simulink model "ENV_old_working"  (R2024b)
settings: Solver=FixedStepDiscrete  StartTime=0.0  StopTime=1  FixedStep=0.001  RelTol=1e-3  EnableMultiTasking=on
libraries: stm32blockslib x68, canmsglib x32, stm32f4xxblockslib x20, simulink x8
(part 3 of 4)

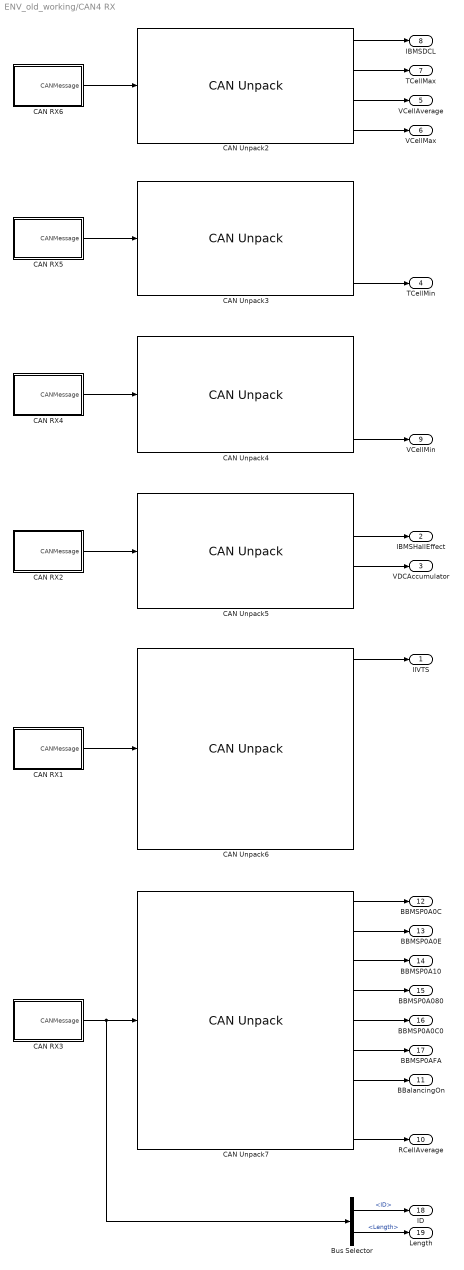
== system ENV_old_working/CAN4 RX ==
  Bus Selector : BusSelector  OutputSignals=ID,Length
  CAN RX1 : Subsystem  mask{SPIModuleSelect=SPI1, Port_Select=GPIOC, Pin=5, PortName=GPIOC, PinNumber=4}
      mask prompts: SPIModuleSelect "SPI Module"; Port_Select "CS Port"; Pin "CS Pin"; PortName "INT Port"; PinNumber "INT Pin"
      mask TypeOptions SPIModuleSelect:
      | Enabled
      | Subsystem/SPI Controller Transfer7/SPIModuleSelect
      mask TypeOptions Port_Select:
      | Enabled
      | Subsystem/SPI Controller Transfer7/Port_Select
      mask TypeOptions Pin:
      | Enabled
      | Subsystem/SPI Controller Transfer7/Pin
      mask TypeOptions PortName: Digital Port Read5/PortName
      mask TypeOptions PinNumber: Digital Port Read5/PinNumber
      mask DialogControl DescTextVar Prompt: Read RX buffer when the INT pin is pulled low. Outputs a CANMessage type to be fed into a CAN unpack
      mask Display:
      | %port_label('output', 1, 'CANMessage');
      | 
      | text(0.05, 0.5, '' + string(get_param(gcb,'SPIModuleSelect')), HorizontalAlignment = 'left');
      | text(0.05, 0.85, 'CS ' + string(get_param(gcb,'Port_Select')) + ' Pin ' + string(get_param(gcb,'Pin')), HorizontalAlignment = 'left');
      | 
      | 
      | text(0.05, 0.15, 'INT ' + string(get_param(gcb,'PortName')) + ' Pin ' + string(get_param(gcb,'PinNumber')), HorizontalAlignment = 'left');
      | %text(0.05, 0.15, 'INT Pin ' + string(get_param(gcb,'PinNumber')), HorizontalAlignment = 'left');
      | 
      | 
      | % OBR logo
      | pos = get_param(gcb, 'Position');
      | blockAspect = (pos(3)-pos(1)) / (pos(4)-pos(2));
      | 
      | % fit(img, m, cx, cy): m = fraction of block the image occupies,
      | % (cx,cy) = center point in normalized 0-1 coords
      | fit = @(img,m,cx,cy) [ ...
      |     cx - m*min(1,(size(img,2)/size(img,1))/blockAspect)/2, ...
      |     cy - m*min(1,blockAspect/(size(img,2)/size(img,1)))/2, ...
      |     m*min(1,(size(img,2)/size(img,1))/blockAspect), ...
      |     m*min(1,blockAspect/(size(img,2)/size(img,1))) ];
      | 
      | ud = get_param(gcb, 'UserData');
      | 
      | image(ud.mcplogo, fit(ud.mcplogo, 0.3, 0.85, 0.5));
      | image(ud.obrlogo, fit(ud.obrlogo, 0.5, 0.5, 0.5));
  CAN RX2 : Subsystem  mask{SPIModuleSelect=SPI1, Port_Select=GPIOC, Pin=5, PortName=GPIOC, PinNumber=4}
      mask prompts: SPIModuleSelect "SPI Module"; Port_Select "CS Port"; Pin "CS Pin"; PortName "INT Port"; PinNumber "INT Pin"
      mask TypeOptions SPIModuleSelect:
      | Enabled
      | Subsystem/SPI Controller Transfer7/SPIModuleSelect
      mask TypeOptions Port_Select:
      | Enabled
      | Subsystem/SPI Controller Transfer7/Port_Select
      mask TypeOptions Pin:
      | Enabled
      | Subsystem/SPI Controller Transfer7/Pin
      mask TypeOptions PortName: Digital Port Read5/PortName
      mask TypeOptions PinNumber: Digital Port Read5/PinNumber
      mask DialogControl DescTextVar Prompt: Read RX buffer when the INT pin is pulled low. Outputs a CANMessage type to be fed into a CAN unpack
      mask Display:
      | %port_label('output', 1, 'CANMessage');
      | 
      | text(0.05, 0.5, '' + string(get_param(gcb,'SPIModuleSelect')), HorizontalAlignment = 'left');
      | text(0.05, 0.85, 'CS ' + string(get_param(gcb,'Port_Select')) + ' Pin ' + string(get_param(gcb,'Pin')), HorizontalAlignment = 'left');
      | 
      | 
      | text(0.05, 0.15, 'INT ' + string(get_param(gcb,'PortName')) + ' Pin ' + string(get_param(gcb,'PinNumber')), HorizontalAlignment = 'left');
      | %text(0.05, 0.15, 'INT Pin ' + string(get_param(gcb,'PinNumber')), HorizontalAlignment = 'left');
      | 
      | 
      | % OBR logo
      | pos = get_param(gcb, 'Position');
      | blockAspect = (pos(3)-pos(1)) / (pos(4)-pos(2));
      | 
      | % fit(img, m, cx, cy): m = fraction of block the image occupies,
      | % (cx,cy) = center point in normalized 0-1 coords
      | fit = @(img,m,cx,cy) [ ...
      |     cx - m*min(1,(size(img,2)/size(img,1))/blockAspect)/2, ...
      |     cy - m*min(1,blockAspect/(size(img,2)/size(img,1)))/2, ...
      |     m*min(1,(size(img,2)/size(img,1))/blockAspect), ...
      |     m*min(1,blockAspect/(size(img,2)/size(img,1))) ];
      | 
      | ud = get_param(gcb, 'UserData');
      | 
      | image(ud.mcplogo, fit(ud.mcplogo, 0.3, 0.85, 0.5));
      | image(ud.obrlogo, fit(ud.obrlogo, 0.5, 0.5, 0.5));
  CAN RX3 : Subsystem  mask{SPIModuleSelect=SPI1, Port_Select=GPIOC, Pin=5, PortName=GPIOC, PinNumber=4}
      mask prompts: SPIModuleSelect "SPI Module"; Port_Select "CS Port"; Pin "CS Pin"; PortName "INT Port"; PinNumber "INT Pin"
      mask TypeOptions SPIModuleSelect:
      | Enabled
      | Subsystem/SPI Controller Transfer7/SPIModuleSelect
      mask TypeOptions Port_Select:
      | Enabled
      | Subsystem/SPI Controller Transfer7/Port_Select
      mask TypeOptions Pin:
      | Enabled
      | Subsystem/SPI Controller Transfer7/Pin
      mask TypeOptions PortName: Digital Port Read5/PortName
      mask TypeOptions PinNumber: Digital Port Read5/PinNumber
      mask DialogControl DescTextVar Prompt: Read RX buffer when the INT pin is pulled low. Outputs a CANMessage type to be fed into a CAN unpack
      mask Display:
      | %port_label('output', 1, 'CANMessage');
      | 
      | text(0.05, 0.5, '' + string(get_param(gcb,'SPIModuleSelect')), HorizontalAlignment = 'left');
      | text(0.05, 0.85, 'CS ' + string(get_param(gcb,'Port_Select')) + ' Pin ' + string(get_param(gcb,'Pin')), HorizontalAlignment = 'left');
      | 
      | 
      | text(0.05, 0.15, 'INT ' + string(get_param(gcb,'PortName')) + ' Pin ' + string(get_param(gcb,'PinNumber')), HorizontalAlignment = 'left');
      | %text(0.05, 0.15, 'INT Pin ' + string(get_param(gcb,'PinNumber')), HorizontalAlignment = 'left');
      | 
      | 
      | % OBR logo
      | pos = get_param(gcb, 'Position');
      | blockAspect = (pos(3)-pos(1)) / (pos(4)-pos(2));
      | 
      | % fit(img, m, cx, cy): m = fraction of block the image occupies,
      | % (cx,cy) = center point in normalized 0-1 coords
      | fit = @(img,m,cx,cy) [ ...
      |     cx - m*min(1,(size(img,2)/size(img,1))/blockAspect)/2, ...
      |     cy - m*min(1,blockAspect/(size(img,2)/size(img,1)))/2, ...
      |     m*min(1,(size(img,2)/size(img,1))/blockAspect), ...
      |     m*min(1,blockAspect/(size(img,2)/size(img,1))) ];
      | 
      | ud = get_param(gcb, 'UserData');
      | 
      | image(ud.mcplogo, fit(ud.mcplogo, 0.3, 0.85, 0.5));
      | image(ud.obrlogo, fit(ud.obrlogo, 0.5, 0.5, 0.5));
  CAN RX4 : Subsystem  mask{SPIModuleSelect=SPI1, Port_Select=GPIOC, Pin=5, PortName=GPIOC, PinNumber=4}
      mask prompts: SPIModuleSelect "SPI Module"; Port_Select "CS Port"; Pin "CS Pin"; PortName "INT Port"; PinNumber "INT Pin"
      mask TypeOptions SPIModuleSelect:
      | Enabled
      | Subsystem/SPI Controller Transfer7/SPIModuleSelect
      mask TypeOptions Port_Select:
      | Enabled
      | Subsystem/SPI Controller Transfer7/Port_Select
      mask TypeOptions Pin:
      | Enabled
      | Subsystem/SPI Controller Transfer7/Pin
      mask TypeOptions PortName: Digital Port Read5/PortName
      mask TypeOptions PinNumber: Digital Port Read5/PinNumber
      mask DialogControl DescTextVar Prompt: Read RX buffer when the INT pin is pulled low. Outputs a CANMessage type to be fed into a CAN unpack
      mask Display:
      | %port_label('output', 1, 'CANMessage');
      | 
      | text(0.05, 0.5, '' + string(get_param(gcb,'SPIModuleSelect')), HorizontalAlignment = 'left');
      | text(0.05, 0.85, 'CS ' + string(get_param(gcb,'Port_Select')) + ' Pin ' + string(get_param(gcb,'Pin')), HorizontalAlignment = 'left');
      | 
      | 
      | text(0.05, 0.15, 'INT ' + string(get_param(gcb,'PortName')) + ' Pin ' + string(get_param(gcb,'PinNumber')), HorizontalAlignment = 'left');
      | %text(0.05, 0.15, 'INT Pin ' + string(get_param(gcb,'PinNumber')), HorizontalAlignment = 'left');
      | 
      | 
      | % OBR logo
      | pos = get_param(gcb, 'Position');
      | blockAspect = (pos(3)-pos(1)) / (pos(4)-pos(2));
      | 
      | % fit(img, m, cx, cy): m = fraction of block the image occupies,
      | % (cx,cy) = center point in normalized 0-1 coords
      | fit = @(img,m,cx,cy) [ ...
      |     cx - m*min(1,(size(img,2)/size(img,1))/blockAspect)/2, ...
      |     cy - m*min(1,blockAspect/(size(img,2)/size(img,1)))/2, ...
      |     m*min(1,(size(img,2)/size(img,1))/blockAspect), ...
      |     m*min(1,blockAspect/(size(img,2)/size(img,1))) ];
      | 
      | ud = get_param(gcb, 'UserData');
      | 
      | image(ud.mcplogo, fit(ud.mcplogo, 0.3, 0.85, 0.5));
      | image(ud.obrlogo, fit(ud.obrlogo, 0.5, 0.5, 0.5));
  CAN RX5 : Subsystem  mask{SPIModuleSelect=SPI1, Port_Select=GPIOC, Pin=5, PortName=GPIOC, PinNumber=4}
      mask prompts: SPIModuleSelect "SPI Module"; Port_Select "CS Port"; Pin "CS Pin"; PortName "INT Port"; PinNumber "INT Pin"
      mask TypeOptions SPIModuleSelect:
      | Enabled
      | Subsystem/SPI Controller Transfer7/SPIModuleSelect
      mask TypeOptions Port_Select:
      | Enabled
      | Subsystem/SPI Controller Transfer7/Port_Select
      mask TypeOptions Pin:
      | Enabled
      | Subsystem/SPI Controller Transfer7/Pin
      mask TypeOptions PortName: Digital Port Read5/PortName
      mask TypeOptions PinNumber: Digital Port Read5/PinNumber
      mask DialogControl DescTextVar Prompt: Read RX buffer when the INT pin is pulled low. Outputs a CANMessage type to be fed into a CAN unpack
      mask Display:
      | %port_label('output', 1, 'CANMessage');
      | 
      | text(0.05, 0.5, '' + string(get_param(gcb,'SPIModuleSelect')), HorizontalAlignment = 'left');
      | text(0.05, 0.85, 'CS ' + string(get_param(gcb,'Port_Select')) + ' Pin ' + string(get_param(gcb,'Pin')), HorizontalAlignment = 'left');
      | 
      | 
      | text(0.05, 0.15, 'INT ' + string(get_param(gcb,'PortName')) + ' Pin ' + string(get_param(gcb,'PinNumber')), HorizontalAlignment = 'left');
      | %text(0.05, 0.15, 'INT Pin ' + string(get_param(gcb,'PinNumber')), HorizontalAlignment = 'left');
      | 
      | 
      | % OBR logo
      | pos = get_param(gcb, 'Position');
      | blockAspect = (pos(3)-pos(1)) / (pos(4)-pos(2));
      | 
      | % fit(img, m, cx, cy): m = fraction of block the image occupies,
      | % (cx,cy) = center point in normalized 0-1 coords
      | fit = @(img,m,cx,cy) [ ...
      |     cx - m*min(1,(size(img,2)/size(img,1))/blockAspect)/2, ...
      |     cy - m*min(1,blockAspect/(size(img,2)/size(img,1)))/2, ...
      |     m*min(1,(size(img,2)/size(img,1))/blockAspect), ...
      |     m*min(1,blockAspect/(size(img,2)/size(img,1))) ];
      | 
      | ud = get_param(gcb, 'UserData');
      | 
      | image(ud.mcplogo, fit(ud.mcplogo, 0.3, 0.85, 0.5));
      | image(ud.obrlogo, fit(ud.obrlogo, 0.5, 0.5, 0.5));
  CAN RX6 : Subsystem  mask{SPIModuleSelect=SPI1, Port_Select=GPIOC, Pin=5, PortName=GPIOC, PinNumber=4}
      mask prompts: SPIModuleSelect "SPI Module"; Port_Select "CS Port"; Pin "CS Pin"; PortName "INT Port"; PinNumber "INT Pin"
      mask TypeOptions SPIModuleSelect:
      | Enabled
      | Subsystem/SPI Controller Transfer7/SPIModuleSelect
      mask TypeOptions Port_Select:
      | Enabled
      | Subsystem/SPI Controller Transfer7/Port_Select
      mask TypeOptions Pin:
      | Enabled
      | Subsystem/SPI Controller Transfer7/Pin
      mask TypeOptions PortName: Digital Port Read5/PortName
      mask TypeOptions PinNumber: Digital Port Read5/PinNumber
      mask DialogControl DescTextVar Prompt: Read RX buffer when the INT pin is pulled low. Outputs a CANMessage type to be fed into a CAN unpack
      mask Display:
      | %port_label('output', 1, 'CANMessage');
      | 
      | text(0.05, 0.5, '' + string(get_param(gcb,'SPIModuleSelect')), HorizontalAlignment = 'left');
      | text(0.05, 0.85, 'CS ' + string(get_param(gcb,'Port_Select')) + ' Pin ' + string(get_param(gcb,'Pin')), HorizontalAlignment = 'left');
      | 
      | 
      | text(0.05, 0.15, 'INT ' + string(get_param(gcb,'PortName')) + ' Pin ' + string(get_param(gcb,'PinNumber')), HorizontalAlignment = 'left');
      | %text(0.05, 0.15, 'INT Pin ' + string(get_param(gcb,'PinNumber')), HorizontalAlignment = 'left');
      | 
      | 
      | % OBR logo
      | pos = get_param(gcb, 'Position');
      | blockAspect = (pos(3)-pos(1)) / (pos(4)-pos(2));
      | 
      | % fit(img, m, cx, cy): m = fraction of block the image occupies,
      | % (cx,cy) = center point in normalized 0-1 coords
      | fit = @(img,m,cx,cy) [ ...
      |     cx - m*min(1,(size(img,2)/size(img,1))/blockAspect)/2, ...
      |     cy - m*min(1,blockAspect/(size(img,2)/size(img,1)))/2, ...
      |     m*min(1,(size(img,2)/size(img,1))/blockAspect), ...
      |     m*min(1,blockAspect/(size(img,2)/size(img,1))) ];
      | 
      | ud = get_param(gcb, 'UserData');
      | 
      | image(ud.mcplogo, fit(ud.mcplogo, 0.3, 0.85, 0.5));
      | image(ud.obrlogo, fit(ud.obrlogo, 0.5, 0.5, 0.5));
  CAN Unpack2 : canmsglib/CAN Unpack  CANdbFile=C:\Users\Will\Desktop\OBR\Embedded\VCUSTM32\Controls\CAN\BMS\26.06.18_CAN4.dbc  MsgList=MSGID_0X6B2  MsgName=MSGID_0X6B2  MsgIDType=Standard (11-bit identifier)  MsgIdentifier=1714  MsgLength=8  SignalInfo={'IBMSDCL','48','16','LE','unsigned','Standard','0','1','0','0','65535';'TCellMax','40','16','BE','signed','Standard','0','1','0','80','32767';'VCellAverage','8','16','BE','unsigned','Standard','0','1e-08','0','0','0.00065535';'VCellMax','24','16','BE','unsigned','Standard','0','0.0001','0','0','6.5535'}  IDPort=off  TimestampPort=off  ErrorPort=off  RemotePort=off  LengthPort=off  StatusPort=off  ApplyMinMax=off
      settings: LibrarySourceBlock=stmutilitieslib/CAN Unpack  DataFormat=CANdb specified signals
  CAN Unpack3 : canmsglib/CAN Unpack  CANdbFile=C:\Users\Will\Desktop\OBR\Embedded\VCUSTM32\Controls\CAN\BMS\26.06.18_CAN4.dbc  MsgList=MSGID_0X6B1  MsgName=MSGID_0X6B1  MsgIDType=Standard (11-bit identifier)  MsgIdentifier=1713  MsgLength=8  SignalInfo={'DTC_Flags_1','16','16','LE','unsigned','Standard','0','1','0','0','65535';'DTC_Flags_2','40','16','BE','unsigned','Standard','0','1','0','0','65535';'Pack_SOC','8','16','BE','unsigned','Standard','0','0.5','0','0','32767.5';'TCellMin','56','16','BE','signed','Standard','0','1','0','80','32767'}  IDPort=off  TimestampPort=off  ErrorPort=off  RemotePort=off  LengthPort=off  StatusPort=off  ApplyMinMax=off
      settings: LibrarySourceBlock=stmutilitieslib/CAN Unpack  DataFormat=CANdb specified signals
  CAN Unpack4 : canmsglib/CAN Unpack  CANdbFile=C:\Users\Will\Desktop\OBR\Embedded\VCUSTM32\Controls\CAN\BMS\26.06.18_CAN4.dbc  MsgList=MSGID_0X6B3  MsgName=MSGID_0X6B3  MsgIDType=Standard (11-bit identifier)  MsgIdentifier=1715  MsgLength=8  SignalInfo={'High_Cell_Resistance','8','16','BE','unsigned','Standard','0','0.01','0','0','655';'Maximum_Cell_Voltage','40','16','BE','unsigned','Standard','0','0.0001','0','0','6.5535';'Minimum_Cell_Voltage','56','16','BE','unsigned','Standard','0','0.0001','0','0','6.5535';'VCellMin','24','16','BE','unsigned','Standard','0','0.0001','0','0','6.5535'}  IDPort=off  TimestampPort=off  ErrorPort=off  RemotePort=off  LengthPort=off  StatusPort=off  ApplyMinMax=off
      settings: LibrarySourceBlock=stmutilitieslib/CAN Unpack  DataFormat=CANdb specified signals
  CAN Unpack5 : canmsglib/CAN Unpack  CANdbFile=C:\Users\Will\Desktop\OBR\Embedded\VCUSTM32\Controls\CAN\BMS\26.06.18_CAN4.dbc  MsgList=MSGID_0X6B0  MsgName=MSGID_0X6B0  MsgIDType=Standard (11-bit identifier)  MsgIdentifier=1712  MsgLength=8  SignalInfo={'CRC_Checksum','48','16','LE','unsigned','Standard','0','1','0','0','65535';'IBMSHallEffect','32','16','LE','signed','Standard','0','1','0','32767','32767';'VDCAccumulator','16','16','LE','unsigned','Standard','0','1','0','0','65535';'VDCAccumulator_NOT','8','16','BE','unsigned','Standard','0','0.1','0','0','6553.5'}  IDPort=off  TimestampPort=off  ErrorPort=off  RemotePort=off  LengthPort=off  StatusPort=off  ApplyMinMax=off
      settings: LibrarySourceBlock=stmutilitieslib/CAN Unpack  DataFormat=CANdb specified signals
  CAN Unpack6 : canmsglib/CAN Unpack  CANdbFile=C:\Users\Will\Desktop\OBR\Embedded\VCUSTM32\Controls\CAN\BMS\26.06.18_CAN4.dbc  MsgList=IVT_Msg_Result_I  MsgName=IVT_Msg_Result_I  MsgIDType=Standard (11-bit identifier)  MsgIdentifier=1313  MsgLength=6  SignalInfo={'IIVTS','40','32','BE','signed','Standard','0','1','0','-2147483648','2147483647';'IVT_ID_Result_I','0','8','BE','unsigned','Standard','0','1','0','0','255';'IVT_MsgCount_Result_I','8','4','BE','unsigned','Standard','0','1','0','0','15';'IVT_Result_I_Channel_Error','13','1','BE','unsigned','Standard','0','1','0','0','1';'IVT_Result_I_Measurement_Error','14','1','BE','unsigned','Standard','0','1','0','0','1';'IVT_Result_I_OCS','12','1','BE','unsigned','Standard','0','1','0','0','1';'IVT_Result_I_System_Error','15','1','BE','unsigned','Standard','0','1','0','0','1'}  IDPort=off  TimestampPort=off  ErrorPort=off  RemotePort=off  LengthPort=off  StatusPort=off  ApplyMinMax=off
      settings: LibrarySourceBlock=stmutilitieslib/CAN Unpack  DataFormat=CANdb specified signals
  CAN Unpack7 : canmsglib/CAN Unpack  CANdbFile=C:\Users\Will\Desktop\OBR\Embedded\VCUSTM32\Controls\CAN\BMS\26.06.18_CAN4.dbc  MsgList=MSGID_0X6B4  MsgName=MSGID_0X6B4  MsgIDType=Standard (11-bit identifier)  MsgIdentifier=1716  MsgLength=8  SignalInfo={'BBMSP0A0C','33','1','LE','unsigned','Standard','0','1','0','0','1';'BBMSP0A0E','34','1','LE','unsigned','Standard','0','1','0','0','1';'BBMSP0A10','35','1','LE','unsigned','Standard','0','1','0','0','1';'BBMSP0A80','36','1','LE','unsigned','Standard','0','1','0','0','1';'BBMSP0AC0','37','1','LE','unsigned','Standard','0','1','0','0','1';'BBMSP0AFA','38','1','LE','unsigned','Standard','0','1','0','0','1';'BBalancingOn','32','1','LE','unsigned','Standard','0','1','0','0','1';'Blank','56','8','LE','unsigned','Standard','0','1','0','0','255';'RCellAverage','8','16','BE','unsigned','Standard','0','0.01','0','0','655'}  IDPort=off  TimestampPort=off  ErrorPort=off  RemotePort=off  LengthPort=off  StatusPort=off  ApplyMinMax=off
      settings: LibrarySourceBlock=stmutilitieslib/CAN Unpack  DataFormat=CANdb specified signals
  IIVTS : Outport  OutDataTypeStr=double
  IBMSHallEffect : Outport  Port=2  OutDataTypeStr=double
  VDCAccumulator : Outport  Port=3  OutDataTypeStr=double
  TCellMin : Outport  Port=4  OutDataTypeStr=double
  VCellAverage : Outport  Port=5  OutDataTypeStr=double
  VCellMax : Outport  Port=6  OutDataTypeStr=double
  TCellMax : Outport  Port=7  OutDataTypeStr=double
  IBMSDCL : Outport  Port=8  OutDataTypeStr=double
  VCellMin : Outport  Port=9  OutDataTypeStr=double
  RCellAverage : Outport  Port=10  OutDataTypeStr=double
  BBalancingOn : Outport  Port=11  OutDataTypeStr=boolean
  BBMSP0A0C : Outport  Port=12  OutDataTypeStr=boolean
  BBMSP0A0E : Outport  Port=13  OutDataTypeStr=boolean
  BBMSP0A10 : Outport  Port=14  OutDataTypeStr=boolean
  BBMSP0A080 : Outport  Port=15  OutDataTypeStr=boolean
  BBMSP0A0C0 : Outport  Port=16  OutDataTypeStr=boolean
  BBMSP0AFA : Outport  Port=17  OutDataTypeStr=boolean
  ID : Outport  Port=18
  Length : Outport  Port=19
  wires:
  Bus Selector/1 -> ID/1  "<ID>"
  Bus Selector/2 -> Length/1  "<Length>"
  CAN Unpack2/1 -> IBMSDCL/1
  CAN Unpack2/2 -> TCellMax/1
  CAN Unpack2/3 -> VCellAverage/1
  CAN Unpack5/2 -> IBMSHallEffect/1
  CAN Unpack6/1 -> IIVTS/1
  CAN Unpack5/3 -> VDCAccumulator/1
  CAN RX6/1(CANMessage) -> CAN Unpack2/1
  CAN RX5/1(CANMessage) -> CAN Unpack3/1
  CAN RX4/1(CANMessage) -> CAN Unpack4/1
  CAN RX2/1(CANMessage) -> CAN Unpack5/1
  CAN RX1/1(CANMessage) -> CAN Unpack6/1
  CAN RX3/1(CANMessage) -> Bus Selector/1, CAN Unpack7/1
  CAN Unpack3/4 -> TCellMin/1
  CAN Unpack2/4 -> VCellMax/1
  CAN Unpack4/4 -> VCellMin/1
  CAN Unpack7/2 -> BBMSP0A0E/1
  CAN Unpack7/3 -> BBMSP0A10/1
  CAN Unpack7/1 -> BBMSP0A0C/1
  CAN Unpack7/9 -> RCellAverage/1
  CAN Unpack7/7 -> BBalancingOn/1
  CAN Unpack7/6 -> BBMSP0AFA/1
  CAN Unpack7/5 -> BBMSP0A0C0/1
  CAN Unpack7/4 -> BBMSP0A080/1

== system ENV_old_working/Initialize CAN1 ==
  Detect Increase : simulink/Logic and Bit Operations/Detect Increase  vinit=0.0  OutDataTypeStr=boolean
  Initialize : Subsystem  TreatAsAtomicUnit=on
  MCPInit : Subsystem  TreatAsAtomicUnit=on
  Step1 : Step
  Step2 : Step
  Unit Delay1 : UnitDelay  SampleTime=-1  HasFrameUpgradeWarning=on
  MCPInitialized : Outport
  wires:
  Detect Increase/1 -> MCPInit/Enable
  Step1/1 -> Detect Increase/1
  Step2/1 -> Unit Delay1/1
  Initialize/1(MCPInitialized) -> MCPInitialized/1
  Unit Delay1/1 -> Initialize/Enable

== system ENV_old_working/Initialize CAN2 ==
  Detect Increase : simulink/Logic and Bit Operations/Detect Increase  vinit=0.0  OutDataTypeStr=boolean
  Initialize : Subsystem  TreatAsAtomicUnit=on
  MCPInit : Subsystem  TreatAsAtomicUnit=on
  Step1 : Step
  Step2 : Step
  Unit Delay1 : UnitDelay  SampleTime=-1  HasFrameUpgradeWarning=on
  MCPInitialized : Outport
  wires:
  Detect Increase/1 -> MCPInit/Enable
  Step1/1 -> Detect Increase/1
  Step2/1 -> Unit Delay1/1
  Initialize/1(MCPInitialized) -> MCPInitialized/1
  Unit Delay1/1 -> Initialize/Enable

== system ENV_old_working/Initialize CAN3 ==
  Detect Increase : simulink/Logic and Bit Operations/Detect Increase  vinit=0.0  OutDataTypeStr=boolean
  Initialize : Subsystem  TreatAsAtomicUnit=on
  MCPInit : Subsystem  TreatAsAtomicUnit=on
  Step1 : Step
  Step2 : Step
  Unit Delay1 : UnitDelay  SampleTime=-1  HasFrameUpgradeWarning=on
  Unit Delay2 : UnitDelay  SampleTime=-1  HasFrameUpgradeWarning=on
  Unit Delay3 : UnitDelay  SampleTime=-1  HasFrameUpgradeWarning=on
  MCPInitialized : Outport
  wires:
  Detect Increase/1 -> MCPInit/Enable
  Step1/1 -> Detect Increase/1
  Step2/1 -> Unit Delay1/1
  Initialize/1(MCPInitialized) -> MCPInitialized/1
  Unit Delay1/1 -> Unit Delay2/1
  Unit Delay2/1 -> Unit Delay3/1
  Unit Delay3/1 -> Initialize/Enable

== system ENV_old_working/Initialize CAN4 ==
  Detect Increase : simulink/Logic and Bit Operations/Detect Increase  vinit=0.0  OutDataTypeStr=boolean
  Initialize : Subsystem  TreatAsAtomicUnit=on
  MCPInit : Subsystem  TreatAsAtomicUnit=on
  Step1 : Step
  Step2 : Step
  Unit Delay1 : UnitDelay  SampleTime=-1  HasFrameUpgradeWarning=on
  Unit Delay2 : UnitDelay  SampleTime=-1  HasFrameUpgradeWarning=on
  Unit Delay3 : UnitDelay  SampleTime=-1  HasFrameUpgradeWarning=on
  MCPInitialized : Outport
  wires:
  Detect Increase/1 -> MCPInit/Enable
  Step1/1 -> Unit Delay3/1
  Step2/1 -> Unit Delay1/1
  Initialize/1(MCPInitialized) -> MCPInitialized/1
  Unit Delay1/1 -> Unit Delay2/1
  Unit Delay2/1 -> Initialize/Enable
  Unit Delay3/1 -> Detect Increase/1

== system ENV_old_working/CAN RX/Enabled Subsystem ==
  Enable : EnablePort
  MATLAB Function7 : MATLAB Function  TreatAsAtomicUnit=on
  Read RX Buffer start at RXB0SIDH7 : Constant  Value=uint8([0x90, 0, 0, 0, 0, 0, 0, 0, 0, 0, 0, 0, 0, 0, 0])
  SPI Controller Transfer7 : stm32blockslib/SPI Controller Transfer  Priority=1  SPIModuleSelect=SPI1  ClockPolarity=Low  ClockPhase=1 Edge  SPIModule=uint32(0)  Mode=Master  BusSpeed=uint32(1000000)  FirstBitToTransfer=Most significant bit (MSB)  ClockMode=0  BlockFunction=Transfer  EnableRegisterAddress=off  RegisterAddress=0  OutputDataType=uint8  OutputDataLength=1  OutputStatus=off  BlockingMode=on  Timeout=0.01  DataBits=8  UseCustomSSPin=Explicit GPIO calls  ActiveLowSSPin=Active low  Port_Select=GPIOB  Pin=Pin
      settings: LibrarySourceBlock=stm32h7xxblockslib/SPI Controller Transfer
  CANMessage : Outport
  wires:
  SPI Controller Transfer7/1 -> MATLAB Function7/1(RxBytes)
  Read RX Buffer start at RXB0SIDH7/1 -> SPI Controller Transfer7/1
  MATLAB Function7/1(Message) -> CANMessage/1

== system ENV_old_working/CAN RX1/Enabled Subsystem ==
  Enable : EnablePort
  MATLAB Function7 : MATLAB Function  TreatAsAtomicUnit=on
  Read RX Buffer start at RXB0SIDH7 : Constant  Value=uint8([0x90, 0, 0, 0, 0, 0, 0, 0, 0, 0, 0, 0, 0, 0, 0])
  SPI Controller Transfer7 : stm32blockslib/SPI Controller Transfer  Priority=1  SPIModuleSelect=SPI1  ClockPolarity=Low  ClockPhase=1 Edge  SPIModule=uint32(0)  Mode=Master  BusSpeed=uint32(1000000)  FirstBitToTransfer=Most significant bit (MSB)  ClockMode=0  BlockFunction=Transfer  EnableRegisterAddress=off  RegisterAddress=0  OutputDataType=uint8  OutputDataLength=1  OutputStatus=off  BlockingMode=on  Timeout=0.01  DataBits=8  UseCustomSSPin=Explicit GPIO calls  ActiveLowSSPin=Active low  Port_Select=GPIOC  Pin=Pin
      settings: LibrarySourceBlock=stm32h7xxblockslib/SPI Controller Transfer
  CANMessage : Outport
  wires:
  SPI Controller Transfer7/1 -> MATLAB Function7/1(RxBytes)
  Read RX Buffer start at RXB0SIDH7/1 -> SPI Controller Transfer7/1
  MATLAB Function7/1(Message) -> CANMessage/1

== system ENV_old_working/CAN RX2/Enabled Subsystem ==
  Enable : EnablePort
  MATLAB Function7 : MATLAB Function  TreatAsAtomicUnit=on
  Read RX Buffer start at RXB0SIDH7 : Constant  Value=uint8([0x90, 0, 0, 0, 0, 0, 0, 0, 0, 0, 0, 0, 0, 0, 0])
  SPI Controller Transfer7 : stm32blockslib/SPI Controller Transfer  Priority=1  SPIModuleSelect=SPI1  ClockPolarity=Low  ClockPhase=1 Edge  SPIModule=uint32(0)  Mode=Master  BusSpeed=uint32(1000000)  FirstBitToTransfer=Most significant bit (MSB)  ClockMode=0  BlockFunction=Transfer  EnableRegisterAddress=off  RegisterAddress=0  OutputDataType=uint8  OutputDataLength=1  OutputStatus=off  BlockingMode=on  Timeout=0.01  DataBits=8  UseCustomSSPin=Explicit GPIO calls  ActiveLowSSPin=Active low  Port_Select=GPIOA  Pin=Pin
      settings: LibrarySourceBlock=stm32h7xxblockslib/SPI Controller Transfer
  CANMessage : Outport
  wires:
  SPI Controller Transfer7/1 -> MATLAB Function7/1(RxBytes)
  Read RX Buffer start at RXB0SIDH7/1 -> SPI Controller Transfer7/1
  MATLAB Function7/1(Message) -> CANMessage/1

== system ENV_old_working/CAN RX3/Enabled Subsystem ==
  Enable : EnablePort
  MATLAB Function7 : MATLAB Function  TreatAsAtomicUnit=on
  Read RX Buffer start at RXB0SIDH7 : Constant  Value=uint8([0x90, 0, 0, 0, 0, 0, 0, 0, 0, 0, 0, 0, 0, 0, 0])
  SPI Controller Transfer7 : stm32blockslib/SPI Controller Transfer  Priority=1  SPIModuleSelect=SPI1  ClockPolarity=Low  ClockPhase=1 Edge  SPIModule=uint32(0)  Mode=Master  BusSpeed=uint32(1000000)  FirstBitToTransfer=Most significant bit (MSB)  ClockMode=0  BlockFunction=Transfer  EnableRegisterAddress=off  RegisterAddress=0  OutputDataType=uint8  OutputDataLength=1  OutputStatus=off  BlockingMode=on  Timeout=0.01  DataBits=8  UseCustomSSPin=Explicit GPIO calls  ActiveLowSSPin=Active low  Port_Select=GPIOC  Pin=Pin
      settings: LibrarySourceBlock=stm32h7xxblockslib/SPI Controller Transfer
  CANMessage : Outport
  wires:
  SPI Controller Transfer7/1 -> MATLAB Function7/1(RxBytes)
  Read RX Buffer start at RXB0SIDH7/1 -> SPI Controller Transfer7/1
  MATLAB Function7/1(Message) -> CANMessage/1

== system ENV_old_working/CAN3 RX/CAN RX ==
  Digital Port Read5 : stm32f4xxblockslib/Digital Port Read  PortName=GPIOA  PinNumber=PinNumber  ReadOperation=on  IOAsArray=off  SampleTime=-1  EnableSimPort=off  hoistedMaskSrc=ECSoC/ECSimCodegen/Digital Port Read
      settings: LibrarySourceBlock=stm32f2xxblockslib/Digital Port Read
  Enabled Subsystem : Subsystem  TreatAsAtomicUnit=on
  NOT5 : Logic  Operator=NOT  IconShape=distinctive  AllPortsSameDT=off  OutDataTypeStr=boolean
  CANMessage : Outport
  wires:
  NOT5/1 -> Enabled Subsystem/Enable
  Digital Port Read5/1 -> NOT5/1
  Enabled Subsystem/1(CANMessage) -> CANMessage/1

== system ENV_old_working/CAN4 RX/CAN RX1 ==
  Digital Port Read5 : stm32f4xxblockslib/Digital Port Read  PortName=GPIOC  PinNumber=PinNumber  ReadOperation=on  IOAsArray=off  SampleTime=-1  EnableSimPort=off  hoistedMaskSrc=ECSoC/ECSimCodegen/Digital Port Read
      settings: LibrarySourceBlock=stm32f2xxblockslib/Digital Port Read
  Enabled Subsystem : Subsystem  TreatAsAtomicUnit=on
  NOT5 : Logic  Operator=NOT  IconShape=distinctive  AllPortsSameDT=off  OutDataTypeStr=boolean
  CANMessage : Outport
  wires:
  NOT5/1 -> Enabled Subsystem/Enable
  Digital Port Read5/1 -> NOT5/1
  Enabled Subsystem/1(CANMessage) -> CANMessage/1

== system ENV_old_working/CAN4 RX/CAN RX2 ==
  Digital Port Read5 : stm32f4xxblockslib/Digital Port Read  PortName=GPIOC  PinNumber=PinNumber  ReadOperation=on  IOAsArray=off  SampleTime=-1  EnableSimPort=off  hoistedMaskSrc=ECSoC/ECSimCodegen/Digital Port Read
      settings: LibrarySourceBlock=stm32f2xxblockslib/Digital Port Read
  Enabled Subsystem : Subsystem  TreatAsAtomicUnit=on
  NOT5 : Logic  Operator=NOT  IconShape=distinctive  AllPortsSameDT=off  OutDataTypeStr=boolean
  CANMessage : Outport
  wires:
  NOT5/1 -> Enabled Subsystem/Enable
  Digital Port Read5/1 -> NOT5/1
  Enabled Subsystem/1(CANMessage) -> CANMessage/1

== system ENV_old_working/CAN4 RX/CAN RX3 ==
  Digital Port Read5 : stm32f4xxblockslib/Digital Port Read  PortName=GPIOC  PinNumber=PinNumber  ReadOperation=on  IOAsArray=off  SampleTime=-1  EnableSimPort=off  hoistedMaskSrc=ECSoC/ECSimCodegen/Digital Port Read
      settings: LibrarySourceBlock=stm32f2xxblockslib/Digital Port Read
  Enabled Subsystem : Subsystem  TreatAsAtomicUnit=on
  NOT5 : Logic  Operator=NOT  IconShape=distinctive  AllPortsSameDT=off  OutDataTypeStr=boolean
  CANMessage : Outport
  wires:
  NOT5/1 -> Enabled Subsystem/Enable
  Digital Port Read5/1 -> NOT5/1
  Enabled Subsystem/1(CANMessage) -> CANMessage/1

== system ENV_old_working/CAN4 RX/CAN RX4 ==
  Digital Port Read5 : stm32f4xxblockslib/Digital Port Read  PortName=GPIOC  PinNumber=PinNumber  ReadOperation=on  IOAsArray=off  SampleTime=-1  EnableSimPort=off  hoistedMaskSrc=ECSoC/ECSimCodegen/Digital Port Read
      settings: LibrarySourceBlock=stm32f2xxblockslib/Digital Port Read
  Enabled Subsystem : Subsystem  TreatAsAtomicUnit=on
  NOT5 : Logic  Operator=NOT  IconShape=distinctive  AllPortsSameDT=off  OutDataTypeStr=boolean
  CANMessage : Outport
  wires:
  NOT5/1 -> Enabled Subsystem/Enable
  Digital Port Read5/1 -> NOT5/1
  Enabled Subsystem/1(CANMessage) -> CANMessage/1

== system ENV_old_working/CAN4 RX/CAN RX5 ==
  Digital Port Read5 : stm32f4xxblockslib/Digital Port Read  PortName=GPIOC  PinNumber=PinNumber  ReadOperation=on  IOAsArray=off  SampleTime=-1  EnableSimPort=off  hoistedMaskSrc=ECSoC/ECSimCodegen/Digital Port Read
      settings: LibrarySourceBlock=stm32f2xxblockslib/Digital Port Read
  Enabled Subsystem : Subsystem  TreatAsAtomicUnit=on
  NOT5 : Logic  Operator=NOT  IconShape=distinctive  AllPortsSameDT=off  OutDataTypeStr=boolean
  CANMessage : Outport
  wires:
  NOT5/1 -> Enabled Subsystem/Enable
  Digital Port Read5/1 -> NOT5/1
  Enabled Subsystem/1(CANMessage) -> CANMessage/1

== system ENV_old_working/CAN4 RX/CAN RX6 ==
  Digital Port Read5 : stm32f4xxblockslib/Digital Port Read  PortName=GPIOC  PinNumber=PinNumber  ReadOperation=on  IOAsArray=off  SampleTime=-1  EnableSimPort=off  hoistedMaskSrc=ECSoC/ECSimCodegen/Digital Port Read
      settings: LibrarySourceBlock=stm32f2xxblockslib/Digital Port Read
  Enabled Subsystem : Subsystem  TreatAsAtomicUnit=on
  NOT5 : Logic  Operator=NOT  IconShape=distinctive  AllPortsSameDT=off  OutDataTypeStr=boolean
  CANMessage : Outport
  wires:
  NOT5/1 -> Enabled Subsystem/Enable
  Digital Port Read5/1 -> NOT5/1
  Enabled Subsystem/1(CANMessage) -> CANMessage/1

== system ENV_old_working/Initialize CAN1/Initialize ==
  Enable : EnablePort
  Constant : Constant  OutDataTypeStr=boolean
  MCPInitialized : Outport
  wires:
  Constant/1 -> MCPInitialized/1

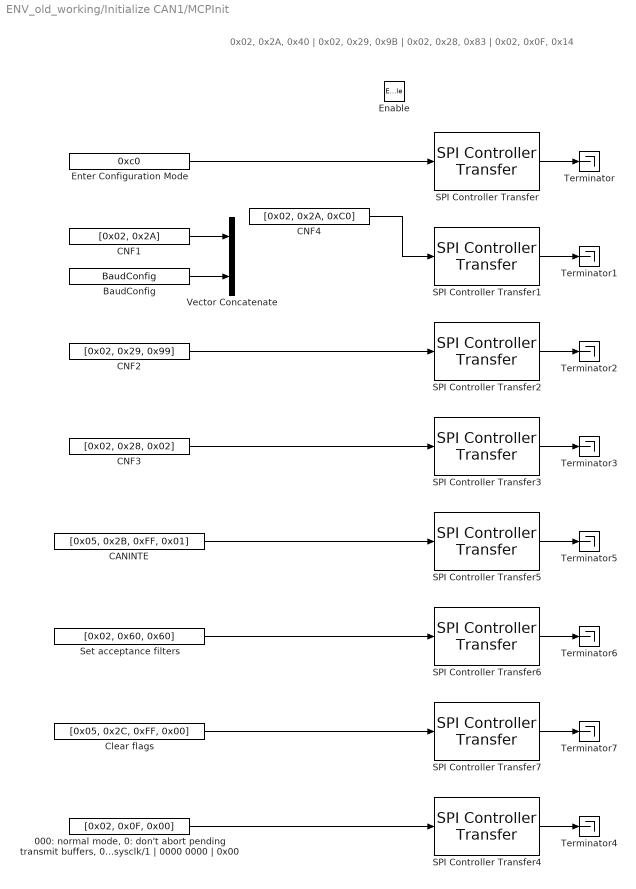
== system ENV_old_working/Initialize CAN1/MCPInit ==
  note: 0x02, 0x2A, 0x40 | 0x02, 0x29, 0x9B | 0x02, 0x28, 0x83 | 0x02, 0x0F, 0x14
  Enable : EnablePort
  " 000: normal mode, 0: don't abort pending transmit buffers, 0: one-shot disabled, 0: CLKOUT disabled, 00: sysclk/1 | 0000 0000 | 0x00" : Constant  Value=[0x02, 0x0F, 0x00]  OutDataTypeStr=uint8
  BaudConfig : Constant  Value=BaudConfig  OutDataTypeStr=uint8
  CANINTE : Constant  Value=[0x05, 0x2B, 0xFF, 0x01]  OutDataTypeStr=uint8
  CNF1 : Constant  Value=[0x02, 0x2A]  OutDataTypeStr=uint8
  CNF2 : Constant  Value=[0x02, 0x29, 0x99]  OutDataTypeStr=uint8
  CNF3 : Constant  Value=[0x02, 0x28, 0x02]  OutDataTypeStr=uint8
  CNF4 : Constant  Value=[0x02, 0x2A, 0xC0]  OutDataTypeStr=uint8
  Clear flags : Constant  Value=[0x05, 0x2C, 0xFF, 0x00]  OutDataTypeStr=uint8
  Enter Configuration Mode : Constant  Value=0xc0  OutDataTypeStr=uint8
  SPI Controller Transfer : stm32blockslib/SPI Controller Transfer  Priority=1  SPIModuleSelect=SPI1  ClockPolarity=Low  ClockPhase=1 Edge  SPIModule=uint32(0)  Mode=Master  BusSpeed=uint32(1000000)  FirstBitToTransfer=Most significant bit (MSB)  ClockMode=0  BlockFunction=Transfer  EnableRegisterAddress=off  RegisterAddress=0  OutputDataType=uint8  OutputDataLength=1  OutputStatus=off  BlockingMode=on  Timeout=0.01  DataBits=8  UseCustomSSPin=Explicit GPIO calls  ActiveLowSSPin=Active low  Port_Select=GPIOB  Pin=Pin
      settings: LibrarySourceBlock=stm32h7xxblockslib/SPI Controller Transfer
  SPI Controller Transfer1 : stm32blockslib/SPI Controller Transfer  Priority=2  SPIModuleSelect=SPI1  ClockPolarity=Low  ClockPhase=1 Edge  SPIModule=uint32(0)  Mode=Master  BusSpeed=uint32(1000000)  FirstBitToTransfer=Most significant bit (MSB)  ClockMode=0  BlockFunction=Transfer  EnableRegisterAddress=off  RegisterAddress=0  OutputDataType=uint8  OutputDataLength=1  OutputStatus=off  BlockingMode=on  Timeout=0.01  DataBits=8  UseCustomSSPin=Explicit GPIO calls  ActiveLowSSPin=Active low  Port_Select=GPIOB  Pin=Pin
      settings: LibrarySourceBlock=stm32h7xxblockslib/SPI Controller Transfer
  SPI Controller Transfer2 : stm32blockslib/SPI Controller Transfer  Priority=3  SPIModuleSelect=SPI1  ClockPolarity=Low  ClockPhase=1 Edge  SPIModule=uint32(0)  Mode=Master  BusSpeed=uint32(1000000)  FirstBitToTransfer=Most significant bit (MSB)  ClockMode=0  BlockFunction=Transfer  EnableRegisterAddress=off  RegisterAddress=0  OutputDataType=uint8  OutputDataLength=1  OutputStatus=off  BlockingMode=on  Timeout=0.01  DataBits=8  UseCustomSSPin=Explicit GPIO calls  ActiveLowSSPin=Active low  Port_Select=GPIOB  Pin=Pin
      settings: LibrarySourceBlock=stm32h7xxblockslib/SPI Controller Transfer
  SPI Controller Transfer3 : stm32blockslib/SPI Controller Transfer  Priority=4  SPIModuleSelect=SPI1  ClockPolarity=Low  ClockPhase=1 Edge  SPIModule=uint32(0)  Mode=Master  BusSpeed=uint32(1000000)  FirstBitToTransfer=Most significant bit (MSB)  ClockMode=0  BlockFunction=Transfer  EnableRegisterAddress=off  RegisterAddress=0  OutputDataType=uint8  OutputDataLength=1  OutputStatus=off  BlockingMode=on  Timeout=0.01  DataBits=8  UseCustomSSPin=Explicit GPIO calls  ActiveLowSSPin=Active low  Port_Select=GPIOB  Pin=Pin
      settings: LibrarySourceBlock=stm32h7xxblockslib/SPI Controller Transfer
  SPI Controller Transfer4 : stm32blockslib/SPI Controller Transfer  Priority=8  SPIModuleSelect=SPI1  ClockPolarity=Low  ClockPhase=1 Edge  SPIModule=uint32(0)  Mode=Master  BusSpeed=uint32(1000000)  FirstBitToTransfer=Most significant bit (MSB)  ClockMode=0  BlockFunction=Transfer  EnableRegisterAddress=off  RegisterAddress=0  OutputDataType=uint8  OutputDataLength=1  OutputStatus=off  BlockingMode=on  Timeout=0.01  DataBits=8  UseCustomSSPin=Explicit GPIO calls  ActiveLowSSPin=Active low  Port_Select=GPIOB  Pin=Pin
      settings: LibrarySourceBlock=stm32h7xxblockslib/SPI Controller Transfer
  SPI Controller Transfer5 : stm32blockslib/SPI Controller Transfer  Priority=5  SPIModuleSelect=SPI1  ClockPolarity=Low  ClockPhase=1 Edge  SPIModule=uint32(0)  Mode=Master  BusSpeed=uint32(1000000)  FirstBitToTransfer=Most significant bit (MSB)  ClockMode=0  BlockFunction=Transfer  EnableRegisterAddress=off  RegisterAddress=0  OutputDataType=uint8  OutputDataLength=1  OutputStatus=off  BlockingMode=on  Timeout=0.01  DataBits=8  UseCustomSSPin=Explicit GPIO calls  ActiveLowSSPin=Active low  Port_Select=GPIOB  Pin=Pin
      settings: LibrarySourceBlock=stm32h7xxblockslib/SPI Controller Transfer
  SPI Controller Transfer6 : stm32blockslib/SPI Controller Transfer  Priority=6  SPIModuleSelect=SPI1  ClockPolarity=Low  ClockPhase=1 Edge  SPIModule=uint32(0)  Mode=Master  BusSpeed=uint32(1000000)  FirstBitToTransfer=Most significant bit (MSB)  ClockMode=0  BlockFunction=Transfer  EnableRegisterAddress=off  RegisterAddress=0  OutputDataType=uint8  OutputDataLength=1  OutputStatus=off  BlockingMode=on  Timeout=0.01  DataBits=8  UseCustomSSPin=Explicit GPIO calls  ActiveLowSSPin=Active low  Port_Select=GPIOB  Pin=Pin
      settings: LibrarySourceBlock=stm32h7xxblockslib/SPI Controller Transfer
  SPI Controller Transfer7 : stm32blockslib/SPI Controller Transfer  Priority=7  SPIModuleSelect=SPI1  ClockPolarity=Low  ClockPhase=1 Edge  SPIModule=uint32(0)  Mode=Master  BusSpeed=uint32(1000000)  FirstBitToTransfer=Most significant bit (MSB)  ClockMode=0  BlockFunction=Transfer  EnableRegisterAddress=off  RegisterAddress=0  OutputDataType=uint8  OutputDataLength=1  OutputStatus=off  BlockingMode=on  Timeout=0.01  DataBits=8  UseCustomSSPin=Explicit GPIO calls  ActiveLowSSPin=Active low  Port_Select=GPIOB  Pin=Pin
      settings: LibrarySourceBlock=stm32h7xxblockslib/SPI Controller Transfer
  Set acceptance filters : Constant  Value=[0x02, 0x60, 0x60]  OutDataTypeStr=uint8
  Terminator{,1..7} (8 alike) : Terminator
  Vector Concatenate : Concatenate
  wires:
  SPI Controller Transfer7/1 -> Terminator7/1
  CNF3/1 -> SPI Controller Transfer3/1
  SPI Controller Transfer6/1 -> Terminator6/1
  CNF2/1 -> SPI Controller Transfer2/1
  CNF4/1 -> SPI Controller Transfer1/1
  SPI Controller Transfer3/1 -> Terminator3/1
  SPI Controller Transfer1/1 -> Terminator1/1
  Clear flags/1 -> SPI Controller Transfer7/1
  SPI Controller Transfer5/1 -> Terminator5/1
  SPI Controller Transfer2/1 -> Terminator2/1
  " 000: normal mode, 0: don't abort pending transmit buffers, 0: one-shot disabled, 0: CLKOUT disabled, 00: sysclk/1 | 0000 0000 | 0x00"/1 -> SPI Controller Transfer4/1
  SPI Controller Transfer4/1 -> Terminator4/1
  CANINTE/1 -> SPI Controller Transfer5/1
  Set acceptance filters/1 -> SPI Controller Transfer6/1
  Enter Configuration Mode/1 -> SPI Controller Transfer/1
  SPI Controller Transfer/1 -> Terminator/1
  BaudConfig/1 -> Vector Concatenate/2
  CNF1/1 -> Vector Concatenate/1

== system ENV_old_working/Initialize CAN2/Initialize ==
  Enable : EnablePort
  Constant : Constant  OutDataTypeStr=boolean
  MCPInitialized : Outport
  wires:
  Constant/1 -> MCPInitialized/1

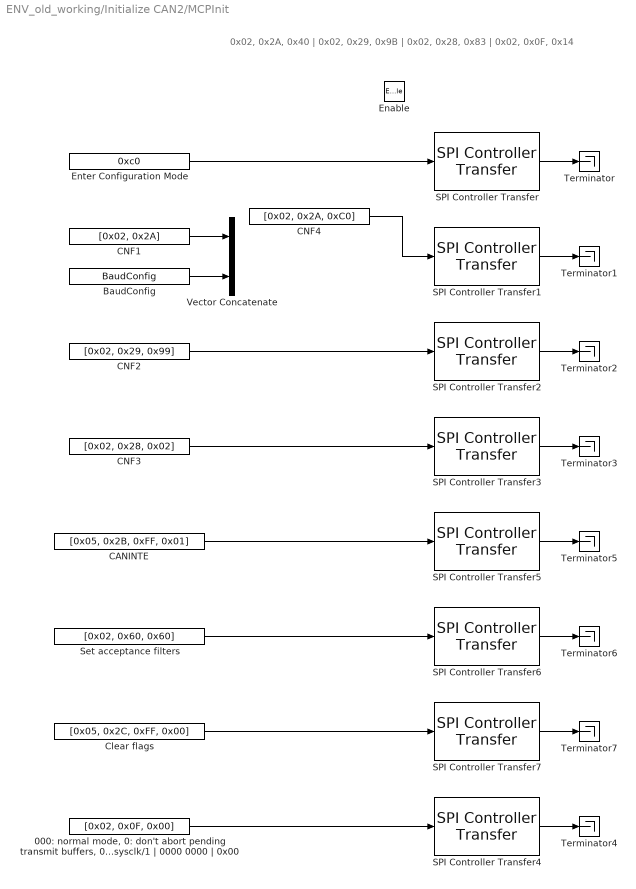
== system ENV_old_working/Initialize CAN2/MCPInit ==
  note: 0x02, 0x2A, 0x40 | 0x02, 0x29, 0x9B | 0x02, 0x28, 0x83 | 0x02, 0x0F, 0x14
  Enable : EnablePort
  " 000: normal mode, 0: don't abort pending transmit buffers, 0: one-shot disabled, 0: CLKOUT disabled, 00: sysclk/1 | 0000 0000 | 0x00" : Constant  Value=[0x02, 0x0F, 0x00]  OutDataTypeStr=uint8
  BaudConfig : Constant  Value=BaudConfig  OutDataTypeStr=uint8
  CANINTE : Constant  Value=[0x05, 0x2B, 0xFF, 0x01]  OutDataTypeStr=uint8
  CNF1 : Constant  Value=[0x02, 0x2A]  OutDataTypeStr=uint8
  CNF2 : Constant  Value=[0x02, 0x29, 0x99]  OutDataTypeStr=uint8
  CNF3 : Constant  Value=[0x02, 0x28, 0x02]  OutDataTypeStr=uint8
  CNF4 : Constant  Value=[0x02, 0x2A, 0xC0]  OutDataTypeStr=uint8
  Clear flags : Constant  Value=[0x05, 0x2C, 0xFF, 0x00]  OutDataTypeStr=uint8
  Enter Configuration Mode : Constant  Value=0xc0  OutDataTypeStr=uint8
  SPI Controller Transfer : stm32blockslib/SPI Controller Transfer  Priority=1  SPIModuleSelect=SPI1  ClockPolarity=Low  ClockPhase=1 Edge  SPIModule=uint32(0)  Mode=Master  BusSpeed=uint32(1000000)  FirstBitToTransfer=Most significant bit (MSB)  ClockMode=0  BlockFunction=Transfer  EnableRegisterAddress=off  RegisterAddress=0  OutputDataType=uint8  OutputDataLength=1  OutputStatus=off  BlockingMode=on  Timeout=0.01  DataBits=8  UseCustomSSPin=Explicit GPIO calls  ActiveLowSSPin=Active low  Port_Select=GPIOC  Pin=Pin
      settings: LibrarySourceBlock=stm32h7xxblockslib/SPI Controller Transfer
  SPI Controller Transfer1 : stm32blockslib/SPI Controller Transfer  Priority=2  SPIModuleSelect=SPI1  ClockPolarity=Low  ClockPhase=1 Edge  SPIModule=uint32(0)  Mode=Master  BusSpeed=uint32(1000000)  FirstBitToTransfer=Most significant bit (MSB)  ClockMode=0  BlockFunction=Transfer  EnableRegisterAddress=off  RegisterAddress=0  OutputDataType=uint8  OutputDataLength=1  OutputStatus=off  BlockingMode=on  Timeout=0.01  DataBits=8  UseCustomSSPin=Explicit GPIO calls  ActiveLowSSPin=Active low  Port_Select=GPIOC  Pin=Pin
      settings: LibrarySourceBlock=stm32h7xxblockslib/SPI Controller Transfer
  SPI Controller Transfer2 : stm32blockslib/SPI Controller Transfer  Priority=3  SPIModuleSelect=SPI1  ClockPolarity=Low  ClockPhase=1 Edge  SPIModule=uint32(0)  Mode=Master  BusSpeed=uint32(1000000)  FirstBitToTransfer=Most significant bit (MSB)  ClockMode=0  BlockFunction=Transfer  EnableRegisterAddress=off  RegisterAddress=0  OutputDataType=uint8  OutputDataLength=1  OutputStatus=off  BlockingMode=on  Timeout=0.01  DataBits=8  UseCustomSSPin=Explicit GPIO calls  ActiveLowSSPin=Active low  Port_Select=GPIOC  Pin=Pin
      settings: LibrarySourceBlock=stm32h7xxblockslib/SPI Controller Transfer
  SPI Controller Transfer3 : stm32blockslib/SPI Controller Transfer  Priority=4  SPIModuleSelect=SPI1  ClockPolarity=Low  ClockPhase=1 Edge  SPIModule=uint32(0)  Mode=Master  BusSpeed=uint32(1000000)  FirstBitToTransfer=Most significant bit (MSB)  ClockMode=0  BlockFunction=Transfer  EnableRegisterAddress=off  RegisterAddress=0  OutputDataType=uint8  OutputDataLength=1  OutputStatus=off  BlockingMode=on  Timeout=0.01  DataBits=8  UseCustomSSPin=Explicit GPIO calls  ActiveLowSSPin=Active low  Port_Select=GPIOC  Pin=Pin
      settings: LibrarySourceBlock=stm32h7xxblockslib/SPI Controller Transfer
  SPI Controller Transfer4 : stm32blockslib/SPI Controller Transfer  Priority=8  SPIModuleSelect=SPI1  ClockPolarity=Low  ClockPhase=1 Edge  SPIModule=uint32(0)  Mode=Master  BusSpeed=uint32(1000000)  FirstBitToTransfer=Most significant bit (MSB)  ClockMode=0  BlockFunction=Transfer  EnableRegisterAddress=off  RegisterAddress=0  OutputDataType=uint8  OutputDataLength=1  OutputStatus=off  BlockingMode=on  Timeout=0.01  DataBits=8  UseCustomSSPin=Explicit GPIO calls  ActiveLowSSPin=Active low  Port_Select=GPIOC  Pin=Pin
      settings: LibrarySourceBlock=stm32h7xxblockslib/SPI Controller Transfer
  SPI Controller Transfer5 : stm32blockslib/SPI Controller Transfer  Priority=5  SPIModuleSelect=SPI1  ClockPolarity=Low  ClockPhase=1 Edge  SPIModule=uint32(0)  Mode=Master  BusSpeed=uint32(1000000)  FirstBitToTransfer=Most significant bit (MSB)  ClockMode=0  BlockFunction=Transfer  EnableRegisterAddress=off  RegisterAddress=0  OutputDataType=uint8  OutputDataLength=1  OutputStatus=off  BlockingMode=on  Timeout=0.01  DataBits=8  UseCustomSSPin=Explicit GPIO calls  ActiveLowSSPin=Active low  Port_Select=GPIOC  Pin=Pin
      settings: LibrarySourceBlock=stm32h7xxblockslib/SPI Controller Transfer
  SPI Controller Transfer6 : stm32blockslib/SPI Controller Transfer  Priority=6  SPIModuleSelect=SPI1  ClockPolarity=Low  ClockPhase=1 Edge  SPIModule=uint32(0)  Mode=Master  BusSpeed=uint32(1000000)  FirstBitToTransfer=Most significant bit (MSB)  ClockMode=0  BlockFunction=Transfer  EnableRegisterAddress=off  RegisterAddress=0  OutputDataType=uint8  OutputDataLength=1  OutputStatus=off  BlockingMode=on  Timeout=0.01  DataBits=8  UseCustomSSPin=Explicit GPIO calls  ActiveLowSSPin=Active low  Port_Select=GPIOC  Pin=Pin
      settings: LibrarySourceBlock=stm32h7xxblockslib/SPI Controller Transfer
  SPI Controller Transfer7 : stm32blockslib/SPI Controller Transfer  Priority=7  SPIModuleSelect=SPI1  ClockPolarity=Low  ClockPhase=1 Edge  SPIModule=uint32(0)  Mode=Master  BusSpeed=uint32(1000000)  FirstBitToTransfer=Most significant bit (MSB)  ClockMode=0  BlockFunction=Transfer  EnableRegisterAddress=off  RegisterAddress=0  OutputDataType=uint8  OutputDataLength=1  OutputStatus=off  BlockingMode=on  Timeout=0.01  DataBits=8  UseCustomSSPin=Explicit GPIO calls  ActiveLowSSPin=Active low  Port_Select=GPIOC  Pin=Pin
      settings: LibrarySourceBlock=stm32h7xxblockslib/SPI Controller Transfer
  Set acceptance filters : Constant  Value=[0x02, 0x60, 0x60]  OutDataTypeStr=uint8
  Terminator{,1..7} (8 alike) : Terminator
  Vector Concatenate : Concatenate
  wires:
  SPI Controller Transfer7/1 -> Terminator7/1
  CNF3/1 -> SPI Controller Transfer3/1
  SPI Controller Transfer6/1 -> Terminator6/1
  CNF2/1 -> SPI Controller Transfer2/1
  CNF4/1 -> SPI Controller Transfer1/1
  SPI Controller Transfer3/1 -> Terminator3/1
  SPI Controller Transfer1/1 -> Terminator1/1
  Clear flags/1 -> SPI Controller Transfer7/1
  SPI Controller Transfer5/1 -> Terminator5/1
  SPI Controller Transfer2/1 -> Terminator2/1
  " 000: normal mode, 0: don't abort pending transmit buffers, 0: one-shot disabled, 0: CLKOUT disabled, 00: sysclk/1 | 0000 0000 | 0x00"/1 -> SPI Controller Transfer4/1
  SPI Controller Transfer4/1 -> Terminator4/1
  CANINTE/1 -> SPI Controller Transfer5/1
  Set acceptance filters/1 -> SPI Controller Transfer6/1
  Enter Configuration Mode/1 -> SPI Controller Transfer/1
  SPI Controller Transfer/1 -> Terminator/1
  BaudConfig/1 -> Vector Concatenate/2
  CNF1/1 -> Vector Concatenate/1

== system ENV_old_working/Initialize CAN3/Initialize ==
  Enable : EnablePort
  Constant : Constant  OutDataTypeStr=boolean
  MCPInitialized : Outport
  wires:
  Constant/1 -> MCPInitialized/1
